simulink model "JoyTrajPlanning"  (R2025b)
settings: Solver=FixedStepAuto  StartTime=0.0  StopTime=inf  FixedStep=1e-3  RelTol=1e-3
model workspace (MAT data in the model file):
  SL_ROS_VariableLengthArrays_MaxSizes.CommonInfo.ArrayTruncateAction = 'EmitWarning'
  SL_ROS_VariableLengthArrays_MaxSizes.MsgTypeMap = containers.Map
  SL_ROS_VariableLengthArrays_MaxSizes.MsgTypeMap.serialization.keys = {'sensor_msgs/JointState'}
  SL_ROS_VariableLengthArrays_MaxSizes.MsgTypeMap.serialization.values{1}(1).PropertyName = 'effort'
  SL_ROS_VariableLengthArrays_MaxSizes.MsgTypeMap.serialization.values{1}(1).DataType = 'double'
  SL_ROS_VariableLengthArrays_MaxSizes.MsgTypeMap.serialization.values{1}(1).MaxLength = 3
  SL_ROS_VariableLengthArrays_MaxSizes.MsgTypeMap.serialization.values{1}(2).PropertyName = 'name'
  SL_ROS_VariableLengthArrays_MaxSizes.MsgTypeMap.serialization.values{1}(2).DataType = 'std_msgs/String'
  SL_ROS_VariableLengthArrays_MaxSizes.MsgTypeMap.serialization.values{1}(2).MaxLength = 16
  SL_ROS_VariableLengthArrays_MaxSizes.MsgTypeMap.serialization.values{1}(3).PropertyName = 'position'
  SL_ROS_VariableLengthArrays_MaxSizes.MsgTypeMap.serialization.values{1}(3).DataType = 'double'
  SL_ROS_VariableLengthArrays_MaxSizes.MsgTypeMap.serialization.values{1}(3).MaxLength = 3
  SL_ROS_VariableLengthArrays_MaxSizes.MsgTypeMap.serialization.values{1}(4).PropertyName = 'velocity'
  SL_ROS_VariableLengthArrays_MaxSizes.MsgTypeMap.serialization.values{1}(4).DataType = 'double'
  SL_ROS_VariableLengthArrays_MaxSizes.MsgTypeMap.serialization.values{1}(4).MaxLength = 3
  SL_ROS_VariableLengthArrays_MaxSizes.MsgTypeMap.serialization.uniformity = 0
  SL_ROS_VariableLengthArrays_MaxSizes.MsgTypeMap.serialization.keyType = 'char'
  SL_ROS_VariableLengthArrays_MaxSizes.MsgTypeMap.serialization.valueType = 'any'
libraries: sl3dlib x1
settings Model: Creator=Asus  LastModifiedBy=Asus
settings OptimizationCC: DefaultParameterBehavior=Inlined  EnhancedBackFolding=on  PassReuseOutputArgsAs=Individual arguments  ZeroExternalMemoryAtStartup=off  ZeroInternalMemoryAtStartup=off  MaxStackSize=64  OptimizeBlockOrder=speed  DifferentSizesBufferReuse=on  OptimizationCustomize=off  EfficientTunableParamExpr=on
settings DebuggingCC: InheritedTsInSrcMsg=none  ParameterTunabilityLossMsg=error
settings SFSimCC: MATLABDynamicMemAlloc=off
settings RTWCC: SystemTargetFile=ert.tlc  HardwareBoard=Robot Operating System 2 (ROS 2)  TLCOptions="-aInlineSetEventsForThisBaseRateFcn=TLC_FALSE -aSuppressMultiTaskScheduler=TLC_FALSE  -aRateBasedStepFcn=0"  TemplateMakefile=ert_default_tmf  Toolchain=Colcon Tools  TargetLang=C++  Description=Embedded Coder
settings CodeAppCC: ForceParamTrailComments=on  IgnoreCustomStorageClasses=off  MaxIdLength=95.0  OperatorAnnotations=on  SimulinkDataObjDesc=on  SFDataObjDesc=on  InsertBlockDesc=on
settings ERTTargetCC: RootIOFormat=Structure reference  CodeInterfacePackaging=C++ class

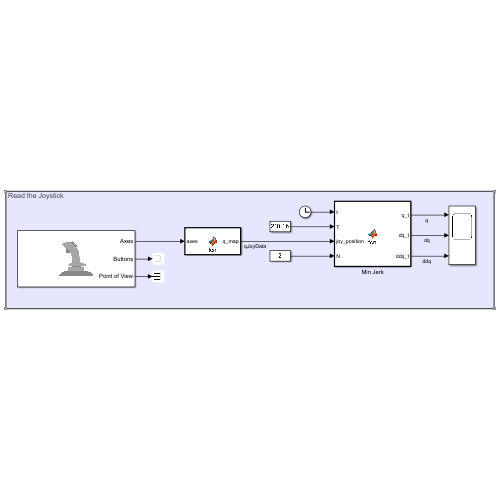
[thumbnail: Simulink's stored preview of the top-level diagram]
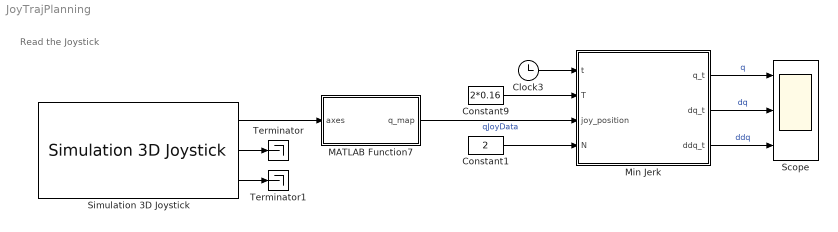
== system JoyTrajPlanning ==
  note: Read the Joystick
  Clock3 : Clock
  Constant1 : Constant  Value=2
  Constant9 : Constant  Value=2*0.16
  MATLAB Function7 : MATLAB Function  TreatAsAtomicUnit=on
  Min Jerk : MATLAB Function  TreatAsAtomicUnit=on
  Scope : Scope  NumInputPorts=3
      settings: ActiveDisplayYMinimum=-1.2480154711471125  ActiveDisplayYMaximum=0.85473834768131374
  Simulation 3D Joystick : sl3dlib/Simulation 3D/Hardware Interface/Simulation 3D Joystick  joyid=1  adjustports=on  forcefeed=off
  Terminator : Terminator
  Terminator1 : Terminator
  wires:
  MATLAB Function7/1(q_map) -> Min Jerk/3(joy_position)  "qJoyData"
  Simulation 3D Joystick/2 -> Terminator/1
  Simulation 3D Joystick/3 -> Terminator1/1
  Clock3/1 -> Min Jerk/1(t)
  Constant9/1 -> Min Jerk/2(T)
  Simulation 3D Joystick/1 -> MATLAB Function7/1(axes)
  Constant1/1 -> Min Jerk/4(N)
  Min Jerk/1(q_t) -> Scope/1  "q"
  Min Jerk/2(dq_t) -> Scope/2  "dq"
  Min Jerk/3(ddq_t) -> Scope/3  "ddq"

== matlab function JoyTrajPlanning/Min Jerk ==
  data: t input; q_t output; T input; joy_position input; dq_t output; ddq_t output; N input
function [q_t, dq_t, ddq_t] = fcn(t, T, joy_position, N)
    %#codegen
    % Sliding-window waypoint planner:
    % - Stores last N joystick positions as waypoints (uniformly spaced by T)
    % - Generates a C2-continuous (pos/vel/acc) quintic segment between wp(:,1)->wp(:,2)
    % - Boundary velocities/accelerations are NOT forced to zero; they are inferred
    %   from the waypoint window (preview) and continuity is enforced by propagating
    %   the end-state of the previous segment.

    % -------- Parameters (adjust maxN if you want bigger buffers) ----------
    maxN = 50;          % compile-time fixed buffer size
    Tmin = 1e-4;        % safety floor for T

    if T < Tmin
        T = Tmin;
    end

    % -------- Persistent state --------------------------------------------
    persistent wp              % 3 x maxN waypoint ring (we'll use first N columns)
    persistent seg_start_time
    persistent x_start dx_start ddx_start
    persistent q_target dq_target ddq_target
    persistent last_T Binv
    persistent initialized

    if isempty(initialized)
        initialized = true;

        % Clamp N to [1,maxN]
        if N < 1
            N = 1;
        elseif N > maxN
            N = maxN;
        end

        % Initialize waypoint buffer: replicate the initial joystick position
        wp = repmat(joy_position, 1, maxN);

        % Initialize segment start at current time
        seg_start_time = t;

        % Start state (you can set x_start=joy_position if you prefer)
        x_start   = wp(:,1);
        dx_start  = zeros(3,1);
        ddx_start = zeros(3,1);

        % Initial target is the "next" waypoint (same initially)
        q_target = wp(:,2);

        % Infer end derivatives from waypoint window (initially zeros)
        [dq_target, ddq_target] = inferEndDerivatives(wp, N, T);

        last_T = -1;
        Binv   = eye(3);
    end

    % Clamp N to [1,maxN] every call (robust to non-const input)
    if N < 1
        N = 1;
    elseif N > maxN
        N = maxN;
    end

    % -------- Cache inverse for this T ------------------------------------
    if isempty(last_T) || (T ~= last_T)
        T2 = T*T;  T3 = T2*T;
        T4 = T3*T; T5 = T4*T;

        b = [ T3,    T4,     T5;
             3*T2,  4*T3,   5*T4;
             6*T,  12*T2, 20*T3 ];

        Binv  = inv(b);
        last_T = T;
    end

    % -------- Segment time -------------------------------------------------
    t_segment = t - seg_start_time;

    % If time advanced past the segment end, advance segments robustly
    while t_segment >= T
        % End state of current segment at t = T (exact, for C2 continuity)
        [x_end, dx_end, ddx_end] = segment3D( ...
            x_start, dx_start, ddx_start, ...
            q_target, dq_target, ddq_target, ...
            T, T, Binv);

        % Promote end state -> new start state (guarantees C2 continuity)
        x_start   = x_end;
        dx_start  = dx_end;
        ddx_start = ddx_end;

        % Shift waypoint window left and append newest joystick sample
        % Use only the first N columns as the active window, but maintain maxN storage
        if N >= 2
            wp(:,1:N-1) = wp(:,2:N);
            wp(:,N)     = joy_position;
        else
            wp(:,1)     = joy_position;
        end

        % New target is next waypoint (wp(:,2)) if available, else current
        if N >= 2
            q_target = wp(:,2);
        else
            q_target = wp(:,1);
        end

        % Infer target end derivatives from waypoint window (no forcing to zero)
        [dq_target, ddq_target] = inferEndDerivatives(wp, N, T);

        % Advance segment start time
        seg_start_time = seg_start_time + T;
        t_segment = t - seg_start_time;
    end

    % Clamp within [0,T] to avoid extrapolation
    if t_segment < 0
        t_segment = 0;
    elseif t_segment > T
        t_segment = T;
    end

    % -------- Compute outputs in current segment ---------------------------
    [q_t, dq_t, ddq_t] = segment3D( ...
        x_start, dx_start, ddx_start, ...
        q_target, dq_target, ddq_target, ...
        T, t_segment, Binv);
end

% =========================================================================
function [dxT, ddxT] = inferEndDerivatives(wp, N, T)
% Estimate velocity/acceleration constraints at the END of the segment
% from the waypoint window (uniformly spaced by T).
%
% We plan from wp(:,1) -> wp(:,2). We infer desired derivatives at wp(:,2).
%
% - If N>=3: central-ish estimates using wp(:,1), wp(:,2), wp(:,3)
% - If N==2: first-difference velocity, zero accel
% - If N==1: zero vel/acc

    dxT  = zeros(3,1);
    ddxT = zeros(3,1);

    if N >= 3
        % Use wp1, wp2, wp3 to infer derivatives at wp2
        p1 = wp(:,1);
        p2 = wp(:,2);
        p3 = wp(:,3);

        % Velocity at p2 (symmetric difference around p2)
        dxT = (p3 - p1) / (2*T);

        % Acceleration at p2 (second difference)
        ddxT = (p3 - 2*p2 + p1) / (T*T);

    elseif N == 2
        p1 = wp(:,1);
        p2 = wp(:,2);

        dxT  = (p2 - p1) / T;
        ddxT = zeros(3,1);

    else
        dxT  = zeros(3,1);
        ddxT = zeros(3,1);
    end
end

% =========================================================================
function [q_t, dq_t, ddq_t] = segment3D(x0, dx0, ddx0, xT, dxT, ddxT, T, t, Binv)
    q_t   = zeros(3,1);
    dq_t  = zeros(3,1);
    ddq_t = zeros(3,1);

    for dim = 1:3
        [q_t(dim), dq_t(dim), ddq_t(dim)] = segment1D( ...
            x0(dim), dx0(dim), ddx0(dim), ...
            xT(dim), dxT(dim), ddxT(dim), ...
            T, t, Binv);
    end
end

% =========================================================================
function [x, dx, ddx] = segment1D(x0, dx0, ddx0, xT, dxT, ddxT, T, t, Binv)
% Quintic meeting (x,dx,ddx) at t=0 and t=T

    T2 = T*T;

    a1 = x0;
    a2 = dx0;
    a3 = ddx0/2;

    c1 = xT  - (a1 + a2*T + a3*T2);
    c2 = dxT - (a2 + 2*a3*T);
    c3 = ddxT - (2*a3);

    a456 = Binv * [c1; c2; c3];
    a4 = a456(1);
    a5 = a456(2);
    a6 = a456(3);

    t2 = t*t;  t3 = t2*t;  t4 = t3*t;  t5 = t4*t;

    x   = a1 + a2*t + a3*t2 + a4*t3 + a5*t4 + a6*t5;
    dx  = a2 + 2*a3*t + 3*a4*t2 + 4*a5*t3 + 5*a6*t4;
    ddx = 2*a3 + 6*a4*t + 12*a5*t2 + 20*a6*t3;
end

== matlab function JoyTrajPlanning/MATLAB Function7 ==
  data: axes input; q_map output
function q_map = fcn(axes)

    q_map = zeros(3, 1);
    scales = [-0.25, 0.5, 1.0];
    q_map(1) = axes(3) * scales(3);
    q_map(2) = axes(2) * scales(2);
    q_map(3) = axes(1) * scales(1);

end
